simulink model "mDriveCycleSrc"  (R2019b)
settings: Solver=ode4  StartTime=0.0  StopTime=1e6  FixedStep=.1  RelTol=1e-3
undefined symbols (not defined in the file): PtbsDriveCycleStructArray, VsrDriveCycleStructArray
libraries: VsrLibDriveCycleSrc x1
settings Model: DataDictionary=DdDriveCycleTest.sldd  EnableAccessToBaseWorkspace=off  SimulationMode=accelerator  Creator=9bt  LastModifiedBy=4qz

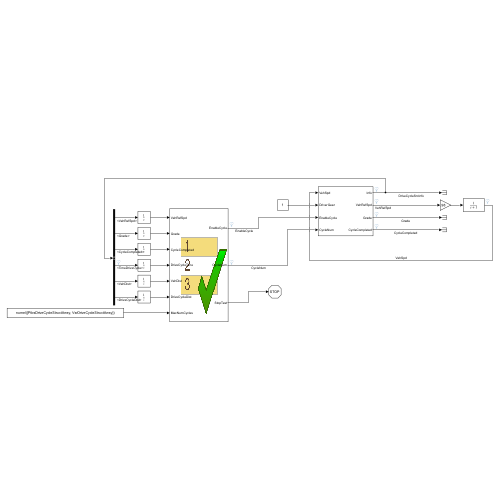
[thumbnail: Simulink's stored preview of the top-level diagram]
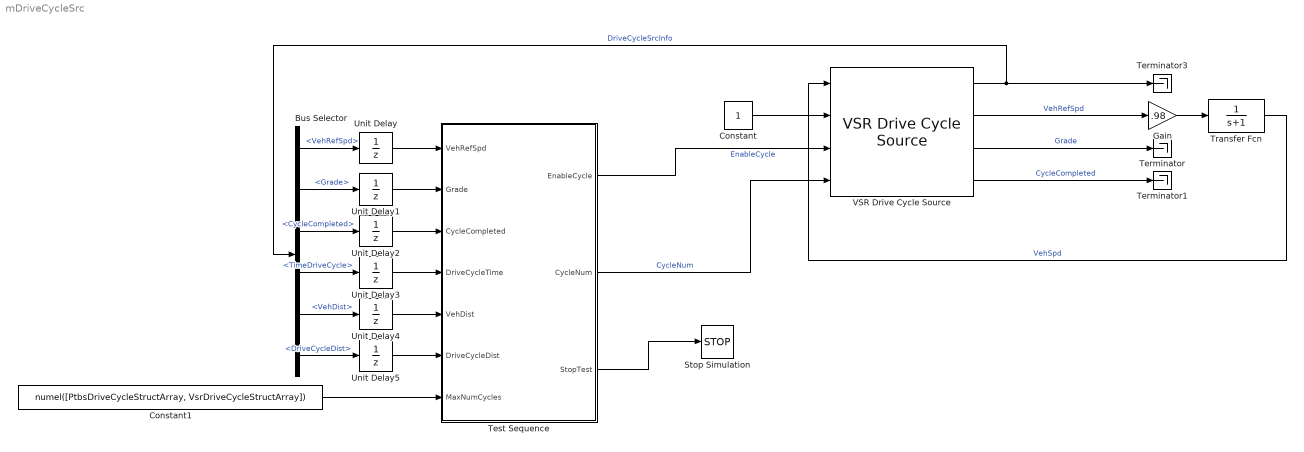
== system mDriveCycleSrc ==
  Bus Selector : BusSelector  OutputSignals=VehRefSpd,Grade,CycleCompleted,TimeDriveCycle,VehDist,DriveCycleDist
  Constant : Constant
  Constant1 : Constant  Value=numel([PtbsDriveCycleStructArray, VsrDriveCycleStructArray])
  Gain : Gain  Gain=.98
  Stop Simulation : Stop
  Terminator : Terminator
  Terminator1 : Terminator
  Terminator3 : Terminator
  Test Sequence : Test Sequence  TreatAsAtomicUnit=on
  Transfer Fcn : TransferFcn  Denominator=[1 1]
  Unit Delay{,1..5} (6 alike) : UnitDelay  SampleTime=-1  HasFrameUpgradeWarning=on
  VSR Drive Cycle Source : VsrLibDriveCycleSrc/VSR Drive Cycle Source  DistCompensationCheckbox=on  DriveCycleStructArray=[PtbsDriveCycleStructArray, VsrDriveCycleStructArray]  TimeLookAhead=0.5
  wires:
  Constant/1 -> VSR Drive Cycle Source/2
  VSR Drive Cycle Source/3 -> Terminator/1  "Grade"
  VSR Drive Cycle Source/4 -> Terminator1/1  "CycleCompleted"
  VSR Drive Cycle Source/2 -> Gain/1  "VehRefSpd"
  VSR Drive Cycle Source/1 -> Bus Selector/1, Terminator3/1  "DriveCycleSrcInfo"
  Test Sequence/1(EnableCycle) -> VSR Drive Cycle Source/3  "EnableCycle"
  Test Sequence/2(CycleNum) -> VSR Drive Cycle Source/4  "CycleNum"
  Bus Selector/1 -> Unit Delay/1  "<VehRefSpd>"
  Bus Selector/2 -> Unit Delay1/1  "<Grade>"
  Bus Selector/3 -> Unit Delay2/1  "<CycleCompleted>"
  Bus Selector/4 -> Unit Delay3/1  "<TimeDriveCycle>"
  Bus Selector/5 -> Unit Delay4/1  "<VehDist>"
  Bus Selector/6 -> Unit Delay5/1  "<DriveCycleDist>"
  Unit Delay/1 -> Test Sequence/1(VehRefSpd)
  Unit Delay1/1 -> Test Sequence/2(Grade)
  Unit Delay2/1 -> Test Sequence/3(CycleCompleted)
  Unit Delay3/1 -> Test Sequence/4(DriveCycleTime)
  Unit Delay4/1 -> Test Sequence/5(VehDist)
  Unit Delay5/1 -> Test Sequence/6(DriveCycleDist)
  Test Sequence/3(StopTest) -> Stop Simulation/1
  Constant1/1 -> Test Sequence/7(MaxNumCycles)
  Transfer Fcn/1 -> VSR Drive Cycle Source/1  "VehSpd"
  Gain/1 -> Transfer Fcn/1

== stateflow chart mDriveCycleSrc/Test Sequence ==
  settings: stateMachineType=SIMPLIFIED_MACHINE
  state Init
    EnableCycle = 0;
    CycleNum = 1;
    CycleIdx = 0;
    StopTest = 0;
  state CheckDisabledCycle
    verify(abs(VehRefSpd) < .001, 'Vehicle reference speed should be 0 when cycle not enabled')
    verify(abs(Grade) < 1e-6, 'Grade should be 0 when cycle not enabled')
  state LoopDriveCycles
    state StartCycle
      CycleIdx = CycleIdx + 1;
      CycleNum = CycleIdx;
      EnableCycle = 1;
    state VerifyDriveCycleTimeAtStart
      verify(DriveCycleTime < 2)
    state WaitToComplete
    state StopCycle
      EnableCycle = 0;
    state VerifyDisabledCycle
      verify(abs(VehRefSpd) < .001, 'Vehicle reference speed should be 0 when cycle not enabled')
      verify(abs(Grade) < 1e-6, 'Grade should be 0 when cycle not enabled')
    (default) -> StartCycle
    (junction 65) -> StartCycle
    (junction 76) -> (junction 65)
    StartCycle -> VerifyDriveCycleTimeAtStart : [
        | true
        | ]
    VerifyDriveCycleTimeAtStart -> WaitToComplete : [
        | after(1, sec)
        | ]
    WaitToComplete -> StopCycle : [
        | CycleCompleted > .99
        | ]
    StopCycle -> VerifyDisabledCycle : [
        | after(.1, sec)
        | ]
    VerifyDisabledCycle -> (junction 76) : [
        | after(1,sec)
        | ]
  state FinishTest
    StopTest = 1;
  (default) -> Init
  Init -> CheckDisabledCycle
  CheckDisabledCycle -> LoopDriveCycles : [
      | after(10,sec)
      | ]
  LoopDriveCycles -> FinishTest : [
      | CycleIdx >= MaxNumCycles
      | ]
  data: EnableCycle output; CycleNum output; VehRefSpd input; Grade input; CycleCompleted input; DriveCycleTime input; VehDist input; DriveCycleDist input; StopTest output size=1; CycleIdx local; MaxNumCycles input
